simulink model "hardware_ekf_est_4para"  (R2020b)
settings: Solver=ode1  StartTime=0.0  StopTime=30  FixedStep=0.01  RelTol=1e-3  EnableMultiTasking=on
libraries: arduinolib x2
settings Model: SILPILModeSetting=veronly  ExtModeTrigDuration=2  Creator=Admin  LastModifiedBy=ONLY-GOD
settings OptimizationCC: EnhancedBackFolding=on  PassReuseOutputArgsAs=Individual arguments  ZeroExternalMemoryAtStartup=off  ZeroInternalMemoryAtStartup=off  MaxStackSize=64  OptimizeBlockOrder=speed  DifferentSizesBufferReuse=on  OptimizationCustomize=off  EfficientTunableParamExpr=on
settings DebuggingCC: ParameterTunabilityLossMsg=error
settings HardwareCC: ProdBitPerPointer=32  ProdBitPerSizeT=32  ProdBitPerPtrDiffT=32  ProdLargestAtomicInteger=Long  ProdLargestAtomicFloat=Double  ProdWordSize=32  ProdHWDeviceType=ARM Compatible->ARM Cortex
settings SFSimCC: MATLABDynamicMemAlloc=off
settings RTWCC: Description=Embedded Coder  SystemTargetFile=ert.tlc  HardwareBoard=Arduino Due  TemplateMakefile=ert_default_tmf  Toolchain=Arduino ARM  BuildConfiguration=Faster Runs
settings CodeAppCC: ForceParamTrailComments=on  IgnoreCustomStorageClasses=off  OperatorAnnotations=on  SimulinkDataObjDesc=on  SFDataObjDesc=on  InsertBlockDesc=on
settings ERTTargetCC: SupportContinuousTime=on  SupportVariableSizeSignals=on  ExtModeTransport=3  ExtModeStaticAllocSize=24576  ExtModeMexFile=ext_xcp  ExtModeIntrfLevel=Level2 - Open

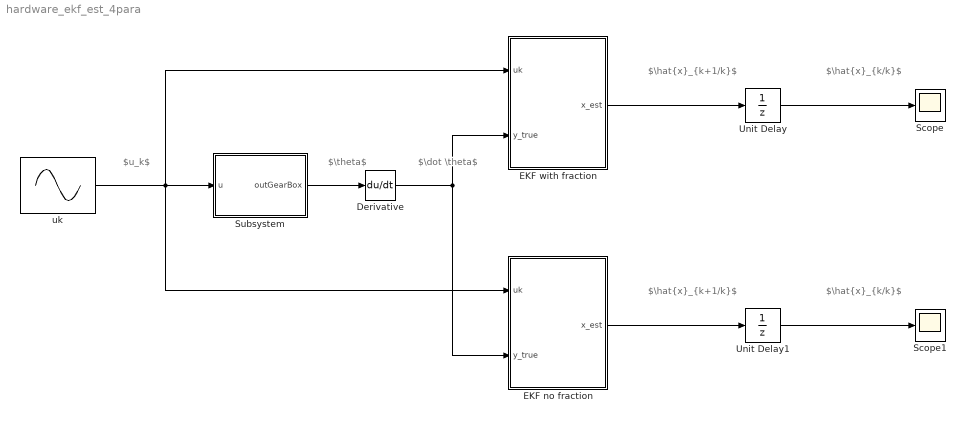
== system hardware_ekf_est_4para ==
  note: $u_k$
  note: $\hat{x}_{k+1/k}$
  note: $\hat{x}_{k/k}$
  note: $\theta$
  note: $\dot \theta$
  note: $\hat{x}_{k+1/k}$
  note: $\hat{x}_{k/k}$
  Derivative : Derivative
  EKF no fraction : MATLAB Function  TreatAsAtomicUnit=on
  EKF with fraction : MATLAB Function  TreatAsAtomicUnit=on
  Scope : Scope
  Scope1 : Scope
  Subsystem : Subsystem
  Unit Delay : UnitDelay  InitialCondition=[0;0;0;0]  SampleTime=-1  HasFrameUpgradeWarning=on
  Unit Delay1 : UnitDelay  InitialCondition=[0;0;0;0]  SampleTime=-1  HasFrameUpgradeWarning=on
  uk : Sin  Amplitude=20  Frequency=2*pi*0.1  SampleTime=0
  wires:
  EKF with fraction/1(x_est) -> Unit Delay/1
  Unit Delay/1 -> Scope/1
  Derivative/1 -> EKF with fraction/2(y_true), EKF no fraction/2(y_true)
  Subsystem/1(outGearBox) -> Derivative/1
  uk/1 -> EKF with fraction/1(uk), Subsystem/1(u), EKF no fraction/1(uk)
  Unit Delay1/1 -> Scope1/1
  EKF no fraction/1(x_est) -> Unit Delay1/1

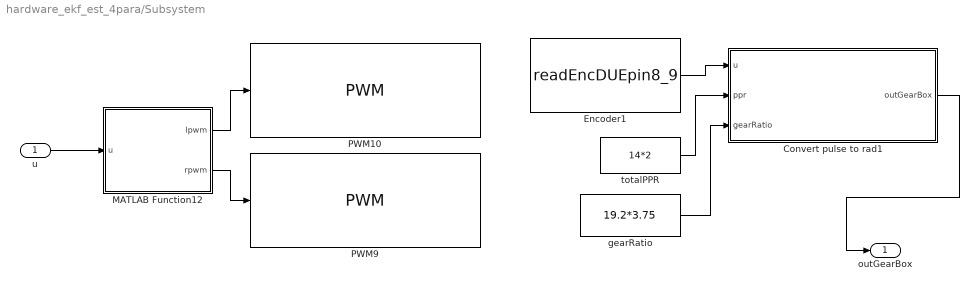
== system hardware_ekf_est_4para/Subsystem ==
  u : Inport
  Convert pulse to rad1 : MATLAB Function  TreatAsAtomicUnit=on
  Encoder1 : S-Function  InitFcn=try, set_param(gcb,'FunctionName','readEncDUEpin8_9'), end  FunctionName=readEncDUEpin8_9  SFunctionModules=readEncDUEpin8_9_wrapper  SFunctionDeploymentMode=off  EnableBusSupport=off  mask(S-Function Builder){}
      mask help: Simulink:masks:SFunctionBuilder_MD
      mask init:
      | val = [[.9  0.75 0.75 1 1 .9 .9 1]',[1 1 0.75 0.75 .9 .9 1 .9]'];try , sys = get_param(gcb,'SfunBuilderFcnName');if isempty(sys), sys = get_param(gcb,'FunctionName'); end,catch, sys = get_param(gcb,'FunctionName'); end
      settings: CopyFcn=set_param(gcbh,'LinkStatus','none')  PreSaveFcn=try, set_param(gcb,'FunctionName','readEncDUEpin8_9'), end  OpenFcn=sfunctionwizard(gcbh)
      mask Display: plot(val(:,1),val(:,2)),disp(sys),port_label('output',1,'count')
  MATLAB Function12 : MATLAB Function  TreatAsAtomicUnit=on
  PWM10 : arduinolib/PWM  pinNumber=7  frequencyType=Default  desiredFrequency=490.2  achievableFrequency=490.2
  PWM9 : arduinolib/PWM  pinNumber=6  frequencyType=Default  desiredFrequency=490.2  achievableFrequency=490.2
  gearRatio : Constant  Value=19.2*3.75
  totalPPR : Constant  Value=14*2
  outGearBox : Outport
  wires:
  Encoder1/1 -> Convert pulse to rad1/1(u)
  MATLAB Function12/1(lpwm) -> PWM10/1
  totalPPR/1 -> Convert pulse to rad1/2(ppr)
  MATLAB Function12/2(rpwm) -> PWM9/1
  gearRatio/1 -> Convert pulse to rad1/3(gearRatio)
  u/1 -> MATLAB Function12/1(u)
  Convert pulse to rad1/1(outGearBox) -> outGearBox/1

== matlab function hardware_ekf_est_4para/EKF with fraction ==
  settings: updateMethod=DISCRETE
  data: uk input; y_true input; x_est output
function x_est = fcn(uk,y_true)
Ts=0.01;
persistent x_est_p P Qd_est R_est Qc_est;
if isempty(x_est_p)
          
          x_est_p=[2;13;25;1];
          P=2*eye(4);
         Qc_est=1e-5*diag([10,25,25,1]);
          Qd_est=Qc_est*Ts;
          R_est=0.02;
end
c=[1 0 0 0];D=0;Ck=c;Dk=D;
%Comput Kalman Gain and update predicted value
Wk=P*Ck'/(Ck*P*Ck'+R_est);
y_est=Ck*x_est_p+Dk*uk;
x=x_est_p+Wk.*(y_true-y_est);
%Compute prediction at next time step
x_est=x+Ts*[-x(2)*x(1)+uk*x(3)-x(4)*sign(x(1));0;0;0];
%Update error covariance matrices
P=P-Wk*Ck*P;
%Define Ak
Ak=eye(4)+Ts*[-x(2) -x(1) uk -sign(x(1));0 0 0 0;0 0 0 0;0 0 0 0];
P=Ak*P*Ak'+Qd_est;
x_est_p=x_est;

== matlab function hardware_ekf_est_4para/EKF no fraction ==
  settings: updateMethod=DISCRETE
  data: uk input; y_true input; x_est output
function x_est = ekf(uk,y_true)
Ts = 0.01;
persistent x_est_p P Qd_est R_est Qc_est;
if isempty(x_est_p)
    x_est_p = [0;0;0];
    P       = 1e-4*diag([10,1,30]);
    Qc_est  = 1e-4*diag([1,10,100]);
    Qd_est  = Ts*Qc_est;
    R_est   = 0.001;
end
c  = [1 0 0];
D  = 0;
Ck = c;
Dk = D;

%Comput Kalman Gain and update predicted value
Wk    = P*Ck'/(Ck*P*Ck'+R_est);
y_est = Ck*x_est_p+Dk*uk;
x     = x_est_p+Wk.*(y_true-y_est);

%Compute prediction at next time step
x_est = x+Ts*[-x(2)*x(1)+uk*x(3);
                          0;
                          0];

%Update error covariance matrices
P = P-Wk*Ck*P;

%Define Ak
Ak      = eye(3)+Ts*[-x(2) -x(1) uk;0 0 0;0 0 0];
P       = Ak*P*Ak'+Qd_est;
x_est_p = x_est;

== matlab function hardware_ekf_est_4para/Subsystem/MATLAB Function12 ==
  data: u input; lpwm output; rpwm output
function [lpwm,rpwm] = fcn(u)

Vmax = 22.9;
pwm = u*254/Vmax;
if pwm > 0
    lpwm = pwm;
    rpwm = 0;
elseif pwm < 0
    lpwm = 0;
    rpwm = abs(pwm);
else
    lpwm = 0;
    rpwm = 0;
end

== matlab function hardware_ekf_est_4para/Subsystem/Convert pulse to rad1 ==
  settings: updateMethod=DISCRETE
  data: u input; ppr input; gearRatio input; outGearBox output
function outGearBox = fcn(u,ppr,gearRatio)

persistent counter_num over_flag
if(isempty(counter_num)), counter_num = 0;end
if(isempty(over_flag)), over_flag = 0;end
pulse2radian = 2*pi/ppr; % 1 pulse = ?? radian

if(double(u) - counter_num > 40000), over_flag = over_flag-1;
elseif(double(u) - counter_num < -40000), over_flag = over_flag+1;
end

inGearBox = (double(u)+over_flag*(2^32 -1))*pulse2radian; 
outGearBox = inGearBox/gearRatio;
counter_num = double(u) ;
